simulink model "suspend_kamotu_kato3"  (R2020b)
settings: Solver=ode15s  StartTime=0.0  StopTime=100  FixedStep=0.0001  MaxStep=0.001
settings Model: Creator=iketa  LastModifiedBy=kt012
settings DebuggingCC: ArithmeticOperatorsInVariantConditions=warning
settings SFSimCC: CustomCodeUndefinedFunction=UseInterfaceOnly

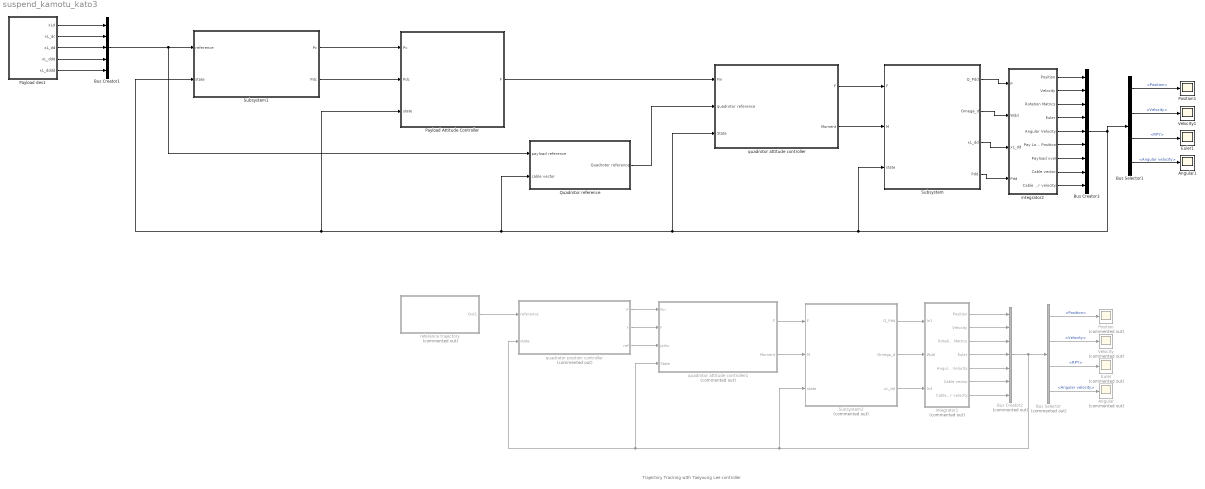
== system suspend_kamotu_kato3 ==
  note: Trajectory Tracking with Taeyoung Lee controller
  Angular : Scope  Commented=on
  Angular1 : Scope
  Bus Creator1 : BusCreator  Inputs=5
  Bus Creator2 : BusCreator  Commented=on  Inputs=7
  Bus Creator3 : BusCreator  Inputs=9
  Bus Selector : BusSelector  Commented=on  OutputSignals=Position,Velocity,RPY,Angular velocity
  Bus Selector1 : BusSelector  OutputSignals=Position,Velocity,RPY,Angular velocity
  Euler : Scope  Commented=on
  Euler1 : Scope
  Payload Attitude Controller : Subsystem
  Payload des1 : MATLAB Function  TreatAsAtomicUnit=on
  Position : Scope  Commented=on
  Position1 : Scope
  Quadrotor reference : Subsystem
  Subsystem : Subsystem
  Subsystem1 : Subsystem
  Subsystem2 : Subsystem  Commented=on
  Velocity : Scope  Commented=on
  Velocity1 : Scope
  integrator1 : Subsystem  Commented=on
  integrator2 : Subsystem
  quadrotor attitude controller : Subsystem
  quadrotor attitude controller1 : Subsystem  Commented=on
  quadrotor position controller : Subsystem  Commented=on
  reference trajectory : Subsystem  Commented=on
  wires:
  Subsystem/1(Q_Pdd) -> integrator2/1(P)
  Subsystem/2(Omega_d) -> integrator2/2(Wdd)
  Subsystem/3(xL_dd) -> integrator2/3(xL_dd)
  Payload Attitude Controller/1(F) -> quadrotor attitude controller/1(Fin)
  quadrotor attitude controller/2(Moment) -> Subsystem/2(M)
  quadrotor attitude controller/1(F) -> Subsystem/1(F)
  Payload des1/4(xL_ddd) -> Bus Creator1/4
  Payload des1/3(xL_dd) -> Bus Creator1/3
  Payload des1/2(xL_dc) -> Bus Creator1/2
  Payload des1/1(xLd) -> Bus Creator1/1
  Bus Creator1/1 -> Quadrotor reference/1(payload reference), Subsystem1/1(reference)
  Subsystem1/1(Pc) -> Payload Attitude Controller/1(Pc)
  Subsystem1/2(Pdc) -> Payload Attitude Controller/2(Pdc)
  quadrotor attitude controller1/1(F) -> Subsystem2/1(F)
  quadrotor attitude controller1/2(Moment) -> Subsystem2/2(M)
  integrator1/6(Cable vector) -> Bus Creator2/6
  integrator1/5(Angular Velocity) -> Bus Creator2/5
  Subsystem2/3(xL_dd) -> integrator1/3(In3)
  integrator1/2(Velocity) -> Bus Creator2/2
  integrator1/3(Rotation Matrics) -> Bus Creator2/3
  Bus Creator2/1 -> quadrotor position controller/2(state), quadrotor attitude controller1/4(State), Subsystem2/3(state), Bus Selector/1
  integrator1/1(Position) -> Bus Creator2/1
  Subsystem2/2(Omega_d) -> integrator1/2(Wdd)
  integrator1/7(Cable vector velocity) -> Bus Creator2/7
  Subsystem2/1(Q_Pdd) -> integrator1/1(In1)
  quadrotor position controller/1(F) -> quadrotor attitude controller1/1(Fin)
  quadrotor position controller/3(ref) -> quadrotor attitude controller1/3(jarkc)
  quadrotor position controller/2(f) -> quadrotor attitude controller1/2(f)
  Bus Selector/1 -> Position/1  "<Position>"
  Bus Selector/2 -> Velocity/1  "<Velocity>"
  Bus Selector/3 -> Euler/1  "<RPY>"
  integrator1/4(Euler) -> Bus Creator2/4
  Bus Selector/4 -> Angular/1  "<Angular velocity>"
  reference trajectory/1(Out1) -> quadrotor position controller/1(reference)
  Payload des1/5(xL_dddd) -> Bus Creator1/5
  Quadrotor reference/1(Quadrotor reference) -> quadrotor attitude controller/2(quadrotor reference)
  Bus Selector1/1 -> Position1/1  "<Position>"
  Bus Selector1/2 -> Velocity1/1  "<Velocity>"
  Bus Selector1/3 -> Euler1/1  "<RPY>"
  Bus Selector1/4 -> Angular1/1  "<Angular velocity>"
  integrator2/4(Euler) -> Bus Creator3/4
  integrator2/2(Velocity) -> Bus Creator3/2
  integrator2/5(Angular Velocity) -> Bus Creator3/5
  integrator2/3(Rotation Matrics) -> Bus Creator3/3
  integrator2/1(Position) -> Bus Creator3/1
  integrator2/9(Cable vector velocity) -> Bus Creator3/9
  Bus Creator3/1 -> Bus Selector1/1, Subsystem/3(state), Subsystem1/2(state), Payload Attitude Controller/3(state), Quadrotor reference/2(cable vector), quadrotor attitude controller/3(State)
  integrator2/8(Cable vector) -> Bus Creator3/8
  Subsystem/4(Pdd) -> integrator2/4(Pdd)
  integrator2/6(Pay Load Position) -> Bus Creator3/6
  integrator2/7(Payload vvel) -> Bus Creator3/7

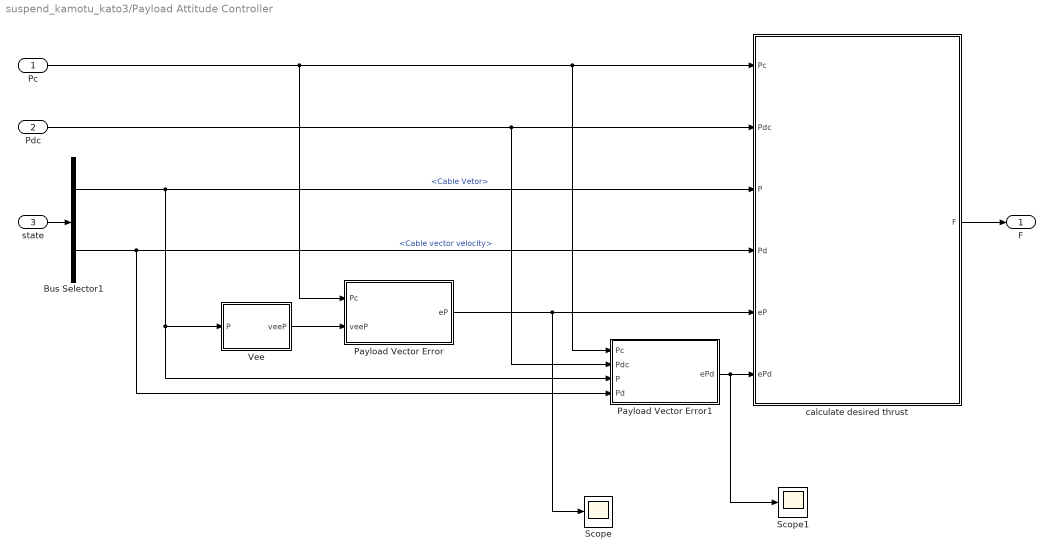
== system suspend_kamotu_kato3/Payload Attitude Controller ==
  Pc : Inport
  Pdc : Inport  Port=2
  state : Inport  Port=3
  Bus Selector1 : BusSelector  OutputSignals=Cable Vetor,Cable vector velocity
  Payload Vector Error : MATLAB Function  TreatAsAtomicUnit=on
  Payload Vector Error1 : MATLAB Function  TreatAsAtomicUnit=on
  Scope : Scope
  Scope1 : Scope
  Vee : MATLAB Function  TreatAsAtomicUnit=on
  calculate desired thrust : MATLAB Function  TreatAsAtomicUnit=on
  F : Outport
  wires:
  Payload Vector Error1/1(ePd) -> Scope1/1, calculate desired thrust/6(ePd)
  state/1 -> Bus Selector1/1
  Pdc/1 -> Payload Vector Error1/2(Pdc), calculate desired thrust/2(Pdc)
  Bus Selector1/1 -> Vee/1(P), Payload Vector Error1/3(P), calculate desired thrust/3(P)  "<Cable Vetor>"
  calculate desired thrust/1(F) -> F/1
  Vee/1(veeP) -> Payload Vector Error/2(veeP)
  Bus Selector1/2 -> Payload Vector Error1/4(Pd), calculate desired thrust/4(Pd)  "<Cable vector velocity>"
  Payload Vector Error/1(eP) -> Scope/1, calculate desired thrust/5(eP)
  Pc/1 -> Payload Vector Error/1(Pc), Payload Vector Error1/1(Pc), calculate desired thrust/1(Pc)

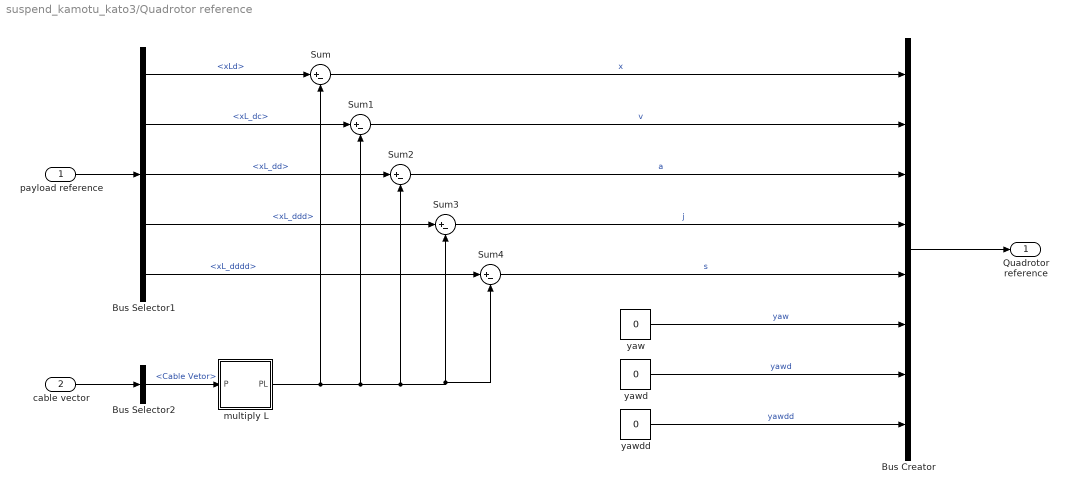
== system suspend_kamotu_kato3/Quadrotor reference ==
  payload reference : Inport
  cable vector : Inport  Port=2
  Bus Creator : BusCreator  Inputs=8
  Bus Selector1 : BusSelector  OutputSignals=xLd,xL_dc,xL_dd,xL_ddd,xL_dddd
  Bus Selector2 : BusSelector  OutputSignals=Cable Vetor
  Sum{,1..4} (5 alike) : Sum  Inputs=|+-
  multiply L : MATLAB Function  TreatAsAtomicUnit=on
  yaw : Constant  Value=0
  yawd : Constant  Value=0
  yawdd : Constant  Value=0
  Quadrotor reference : Outport
  wires:
  Bus Selector1/2 -> Sum1/1  "<xL_dc>"
  multiply L/1(PL) -> Sum4/2, Sum3/2, Sum2/2, Sum1/2, Sum/2
  Sum1/1 -> Bus Creator/2  "v"
  cable vector/1 -> Bus Selector2/1
  Bus Selector1/4 -> Sum3/1  "<xL_ddd>"
  Bus Selector1/1 -> Sum/1  "<xLd>"
  payload reference/1 -> Bus Selector1/1
  Bus Selector1/5 -> Sum4/1  "<xL_dddd>"
  Bus Selector1/3 -> Sum2/1  "<xL_dd>"
  Bus Selector2/1 -> multiply L/1(P)  "<Cable Vetor>"
  Sum2/1 -> Bus Creator/3  "a"
  Sum/1 -> Bus Creator/1  "x"
  Sum3/1 -> Bus Creator/4  "j"
  Sum4/1 -> Bus Creator/5  "s"
  Bus Creator/1 -> Quadrotor reference/1
  yaw/1 -> Bus Creator/6  "yaw"
  yawd/1 -> Bus Creator/7  "yawd"
  yawdd/1 -> Bus Creator/8  "yawdd"

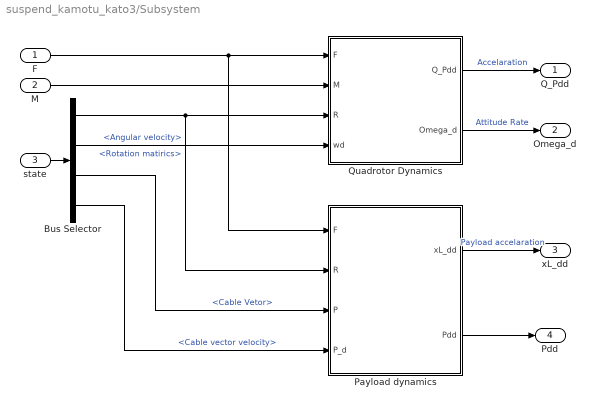
== system suspend_kamotu_kato3/Subsystem ==
  F : Inport
  M : Inport  Port=2
  state : Inport  Port=3
  Bus Selector : BusSelector  OutputSignals=Rotation matirics,Angular velocity,Cable Vetor,Cable vector velocity
  Payload dynamics : MATLAB Function  TreatAsAtomicUnit=on
  Quadrotor Dynamics : MATLAB Function  TreatAsAtomicUnit=on
  Q_Pdd : Outport
  Omega_d : Outport  Port=2
  xL_dd : Outport  Port=3
  Pdd : Outport  Port=4
  wires:
  Payload dynamics/1(xL_dd) -> xL_dd/1  "Payload accelaration"
  Bus Selector/3 -> Payload dynamics/3(P)  "<Cable Vetor>"
  F/1 -> Quadrotor Dynamics/1(F), Payload dynamics/1(F)
  Quadrotor Dynamics/2(Omega_d) -> Omega_d/1  "Attitude Rate"
  Quadrotor Dynamics/1(Q_Pdd) -> Q_Pdd/1  "Accelaration"
  state/1 -> Bus Selector/1
  Bus Selector/1 -> Quadrotor Dynamics/3(R), Payload dynamics/2(R)  "<Rotation matirics>"
  Bus Selector/4 -> Payload dynamics/4(P_d)  "<Cable vector velocity>"
  M/1 -> Quadrotor Dynamics/2(M)
  Bus Selector/2 -> Quadrotor Dynamics/4(wd)  "<Angular velocity>"
  Payload dynamics/2(Pdd) -> Pdd/1

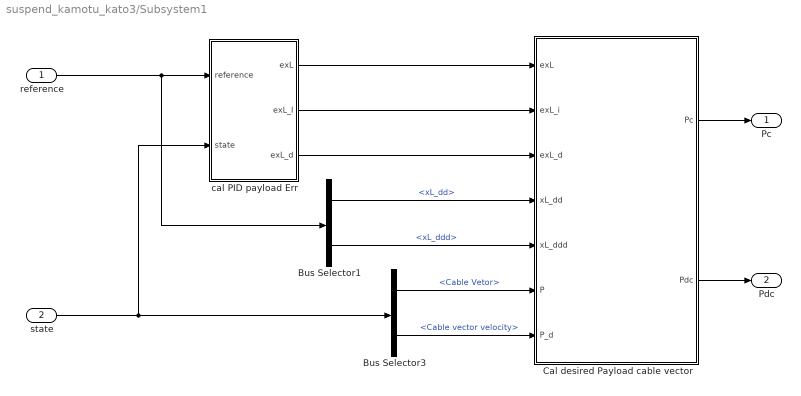
== system suspend_kamotu_kato3/Subsystem1 ==
  reference : Inport
  state : Inport  Port=2
  Bus Selector1 : BusSelector  OutputSignals=xL_dd,xL_ddd
  Bus Selector3 : BusSelector  OutputSignals=Cable Vetor,Cable vector velocity
  Cal desired Payload cable vector : MATLAB Function  TreatAsAtomicUnit=on
  cal PID payload Err : Subsystem
  Pc : Outport
  Pdc : Outport  Port=2
  wires:
  state/1 -> Bus Selector3/1, cal PID payload Err/2(state)
  Bus Selector3/2 -> Cal desired Payload cable vector/7(P_d)  "<Cable vector velocity>"
  Bus Selector3/1 -> Cal desired Payload cable vector/6(P)  "<Cable Vetor>"
  Cal desired Payload cable vector/1(Pc) -> Pc/1
  Cal desired Payload cable vector/2(Pdc) -> Pdc/1
  reference/1 -> Bus Selector1/1, cal PID payload Err/1(reference)
  cal PID payload Err/1(exL) -> Cal desired Payload cable vector/1(exL)
  cal PID payload Err/2(exL_I) -> Cal desired Payload cable vector/2(exL_i)
  cal PID payload Err/3(exL_d) -> Cal desired Payload cable vector/3(exL_d)
  Bus Selector1/1 -> Cal desired Payload cable vector/4(xL_dd)  "<xL_dd>"
  Bus Selector1/2 -> Cal desired Payload cable vector/5(xL_ddd)  "<xL_ddd>"

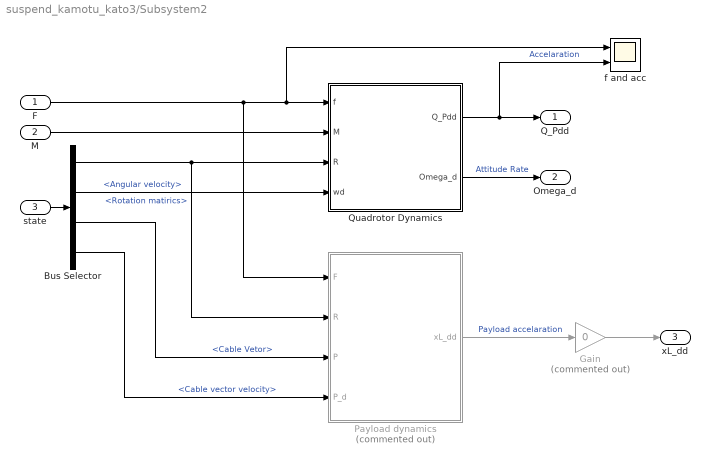
== system suspend_kamotu_kato3/Subsystem2 ==
  F : Inport
  M : Inport  Port=2
  state : Inport  Port=3
  Bus Selector : BusSelector  OutputSignals=Rotation matirics,Angular velocity,Cable Vetor,Cable vector velocity
  Gain : Gain  Commented=on  Gain=0
  Payload dynamics : MATLAB Function  Commented=on  TreatAsAtomicUnit=on
  Quadrotor Dynamics : MATLAB Function  TreatAsAtomicUnit=on
  f and acc : Scope  NumInputPorts=2
  Q_Pdd : Outport
  Omega_d : Outport  Port=2
  xL_dd : Outport  Port=3
  wires:
  Payload dynamics/1(xL_dd) -> Gain/1  "Payload accelaration"
  Bus Selector/3 -> Payload dynamics/3(P)  "<Cable Vetor>"
  F/1 -> Payload dynamics/1(F), f and acc/1, Quadrotor Dynamics/1(f)
  Quadrotor Dynamics/2(Omega_d) -> Omega_d/1  "Attitude Rate"
  Quadrotor Dynamics/1(Q_Pdd) -> f and acc/2, Q_Pdd/1  "Accelaration"
  state/1 -> Bus Selector/1
  Bus Selector/1 -> Payload dynamics/2(R), Quadrotor Dynamics/3(R)  "<Rotation matirics>"
  Bus Selector/4 -> Payload dynamics/4(P_d)  "<Cable vector velocity>"
  M/1 -> Quadrotor Dynamics/2(M)
  Bus Selector/2 -> Quadrotor Dynamics/4(wd)  "<Angular velocity>"
  Gain/1 -> xL_dd/1

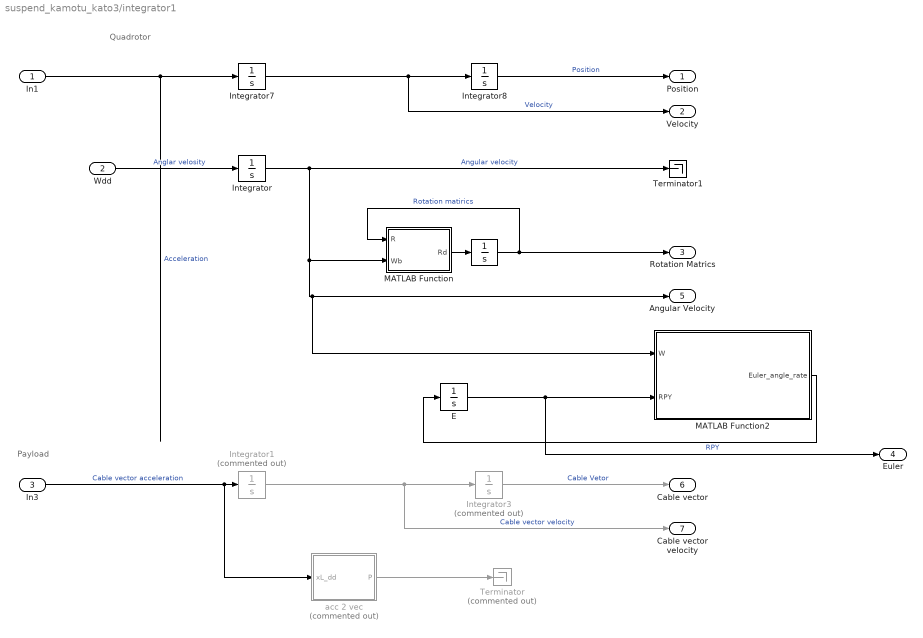
== system suspend_kamotu_kato3/integrator1 ==
  note: Quadrotor
  note: Payload
  In1 : Inport
  Wdd : Inport  Port=2
  In3 : Inport  Port=3
  " " : Integrator  InitialCondition=[1 0 0; 0 1 0; 0 0 1];  ContinuousStateAttributes="\"\""
  E : Integrator  InitialCondition=[0 0 0];
  Integrator : Integrator  InitialCondition=[0 ;0;0];
  Integrator1 : Integrator  Commented=on  InitialCondition=[0;0;0]
  Integrator3 : Integrator  Commented=on  InitialCondition=[0;0;-1]
  Integrator7 : Integrator  InitialCondition=[0;0;0]
  Integrator8 : Integrator  InitialCondition=[0;0;0];
  MATLAB Function : MATLAB Function  TreatAsAtomicUnit=on
  MATLAB Function2 : MATLAB Function  TreatAsAtomicUnit=on
  Terminator : Terminator  Commented=on
  Terminator1 : Terminator
  acc 2 vec : MATLAB Function  Commented=on  TreatAsAtomicUnit=on
  Position : Outport
  Velocity : Outport  Port=2
  Rotation Matrics : Outport  Port=3
  Euler : Outport  Port=4
  Angular Velocity : Outport  Port=5
  Cable vector : Outport  Port=6
  Cable vector velocity : Outport  Port=7
  wires:
  In3/1 -> Integrator1/1, acc 2 vec/1(xL_dd)  "Cable vector acceleration"
  Integrator1/1 -> Integrator3/1, Cable vector velocity/1  "Cable vector velocity"
  acc 2 vec/1(P) -> Terminator/1
  Integrator3/1 -> Cable vector/1  "Cable Vetor"
  Integrator7/1 -> Velocity/1, Integrator8/1  "Velocity"
  Integrator8/1 -> Position/1  "Position"
  In1/1 -> Integrator7/1  "Acceleration"
  MATLAB Function/1(Rd) -> " "/1
  Wdd/1 -> Integrator/1  "Anglar velosity"
  " "/1 -> Rotation Matrics/1, MATLAB Function/1(R)  "Rotation matirics"
  Integrator/1 -> MATLAB Function/2(Wb), MATLAB Function2/1(W), Angular Velocity/1, Terminator1/1  "Angular velocity"
  E/1 -> MATLAB Function2/2(RPY), Euler/1  "RPY"
  MATLAB Function2/1(Euler_angle_rate) -> E/1

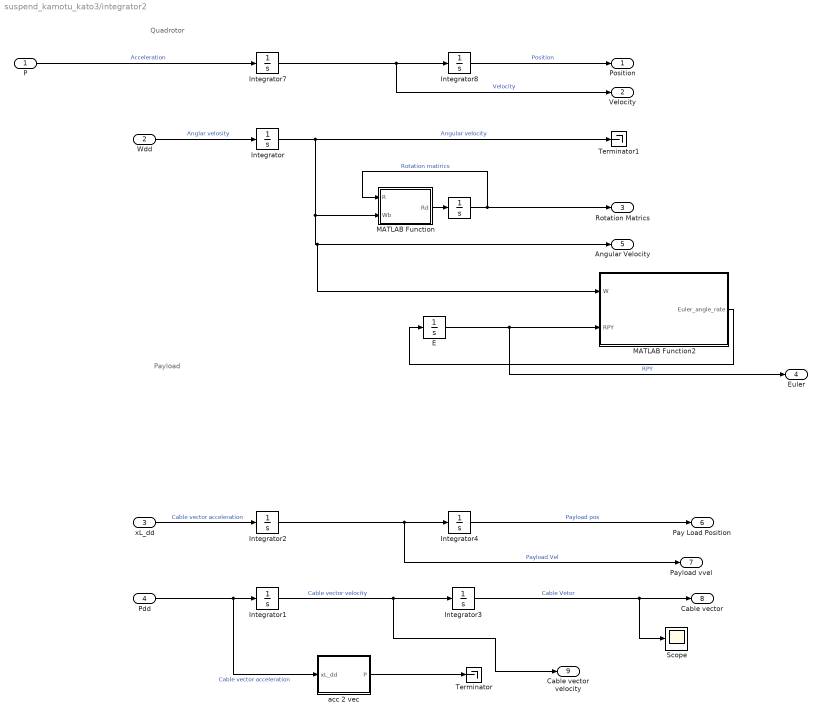
== system suspend_kamotu_kato3/integrator2 ==
  note: Quadrotor
  note: Payload
  P : Inport
  Wdd : Inport  Port=2
  xL_dd : Inport  Port=3
  Pdd : Inport  Port=4
  " " : Integrator  InitialCondition=[1 0 0; 0 1 0; 0 0 1];  ContinuousStateAttributes="\"\""
  E : Integrator  InitialCondition=[0 0 0];
  Integrator : Integrator  InitialCondition=[0 ;0;0];
  Integrator1 : Integrator  InitialCondition=[0;0;0]
  Integrator2 : Integrator  InitialCondition=[0;0;0]
  Integrator3 : Integrator  InitialCondition=[0;0;-1]
  Integrator4 : Integrator  InitialCondition=[0;0;-1]
  Integrator7 : Integrator  InitialCondition=[0;0;0]
  Integrator8 : Integrator  InitialCondition=[0;0;0.1];
  MATLAB Function : MATLAB Function  TreatAsAtomicUnit=on
  MATLAB Function2 : MATLAB Function  TreatAsAtomicUnit=on
  Scope : Scope
  Terminator : Terminator
  Terminator1 : Terminator
  acc 2 vec : MATLAB Function  TreatAsAtomicUnit=on
  Position : Outport
  Velocity : Outport  Port=2
  Rotation Matrics : Outport  Port=3
  Euler : Outport  Port=4
  Angular Velocity : Outport  Port=5
  Pay Load Position : Outport  Port=6
  Payload vvel : Outport  Port=7
  Cable vector : Outport  Port=8
  Cable vector velocity : Outport  Port=9
  wires:
  Pdd/1 -> acc 2 vec/1(xL_dd), Integrator1/1  "Cable vector acceleration"
  Integrator1/1 -> Integrator3/1, Cable vector velocity/1  "Cable vector velocity"
  acc 2 vec/1(P) -> Terminator/1
  Integrator3/1 -> Scope/1, Cable vector/1  "Cable Vetor"
  Integrator7/1 -> Velocity/1, Integrator8/1  "Velocity"
  Integrator8/1 -> Position/1  "Position"
  P/1 -> Integrator7/1  "Acceleration"
  MATLAB Function/1(Rd) -> " "/1
  Wdd/1 -> Integrator/1  "Anglar velosity"
  " "/1 -> Rotation Matrics/1, MATLAB Function/1(R)  "Rotation matirics"
  Integrator/1 -> MATLAB Function/2(Wb), MATLAB Function2/1(W), Angular Velocity/1, Terminator1/1  "Angular velocity"
  E/1 -> MATLAB Function2/2(RPY), Euler/1  "RPY"
  MATLAB Function2/1(Euler_angle_rate) -> E/1
  xL_dd/1 -> Integrator2/1  "Cable vector acceleration"
  Integrator2/1 -> Payload vvel/1, Integrator4/1  "Payload Vel"
  Integrator4/1 -> Pay Load Position/1  "Payload pos"

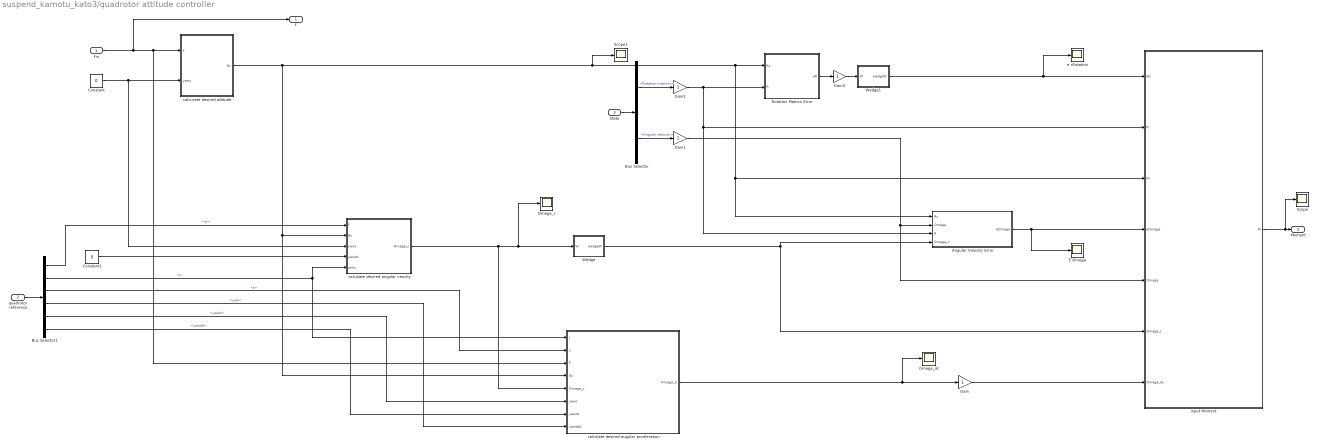
== system suspend_kamotu_kato3/quadrotor attitude controller ==
  Fin : Inport
  quadrotor reference : Inport  Port=2
  State : Inport  Port=3
  Angular Velocity Error : MATLAB Function  TreatAsAtomicUnit=on
  Bus Selector : BusSelector  OutputSignals=Rotation matirics,Angular velocity
  Bus Selector1 : BusSelector  OutputSignals=a,j,s,yaw,yawd,yawdd
  Constant : Constant  Value=0
  Constant1 : Constant  Value=0
  E Omega : Scope
  Gain{,1..3} (4 alike) : Gain
  Omega_c : Scope
  Omega_dc : Scope
  Rotation Matrics Error : MATLAB Function  TreatAsAtomicUnit=on
  Scope : Scope
  Scope1 : Scope
  Wedge : MATLAB Function  TreatAsAtomicUnit=on
  Wedge1 : MATLAB Function  TreatAsAtomicUnit=on
  calculate desired angular veocity : MATLAB Function  TreatAsAtomicUnit=on
  calculate desired augular acceleration : MATLAB Function  TreatAsAtomicUnit=on
  calcurate desired attitude : MATLAB Function  TreatAsAtomicUnit=on
  e rRotation : Scope
  input Moment : MATLAB Function  TreatAsAtomicUnit=on
  F : Outport
  Moment : Outport  Port=2
  wires:
  Gain3/1 -> Wedge1/1(W)
  Gain2/1 -> Angular Velocity Error/3(R), input Moment/2(R), Rotation Matrics Error/2(R)
  Wedge/1(wedgeW) -> Angular Velocity Error/4(Omega_c), input Moment/6(Omega_c)
  calculate desired augular acceleration/1(Omega_d) -> Omega_dc/1, Gain/1
  calculate desired angular veocity/1(Omega_c) -> Omega_c/1, Wedge/1(W), calculate desired augular acceleration/5(Omega_c)
  input Moment/1(M) -> Scope/1, Moment/1
  Bus Selector1/5 -> calculate desired augular acceleration/6(yawc)  "<yawd>"
  Rotation Matrics Error/1(eR) -> Gain3/1
  Gain/1 -> input Moment/7(Omega_dc)
  Bus Selector1/1 -> calculate desired angular veocity/1(F)  "<a>"
  Bus Selector1/4 -> calculate desired augular acceleration/8(yawddc)  "<yaw>"
  Bus Selector1/3 -> calculate desired augular acceleration/2(s)  "<s>"
  Bus Selector/1 -> Gain2/1  "<Rotation matirics>"
  quadrotor reference/1 -> Bus Selector1/1
  State/1 -> Bus Selector/1
  calcurate desired attitude/1(Rc) -> calculate desired augular acceleration/4(Rc), calculate desired angular veocity/2(Rc), Angular Velocity Error/1(Rc), input Moment/3(Rc), Rotation Matrics Error/1(Rc), Scope1/1
  Bus Selector1/6 -> calculate desired augular acceleration/7(yawdc)  "<yawdd>"
  Fin/1 -> F/1, calculate desired augular acceleration/3(F), calcurate desired attitude/1(F)
  Bus Selector1/2 -> calculate desired angular veocity/5(jarkc), calculate desired augular acceleration/1(j)  "<j>"
  Constant/1 -> calcurate desired attitude/2(yawc), calculate desired angular veocity/3(yawc)
  Constant1/1 -> calculate desired angular veocity/4(yawdc)
  Bus Selector/2 -> Gain1/1  "<Angular velocity>"
  Wedge1/1(wedgeW) -> e rRotation/1, input Moment/1(eR)
  Gain1/1 -> input Moment/5(Omega), Angular Velocity Error/2(Omega)
  Angular Velocity Error/1(eOmega) -> E Omega/1, input Moment/4(eOmega)

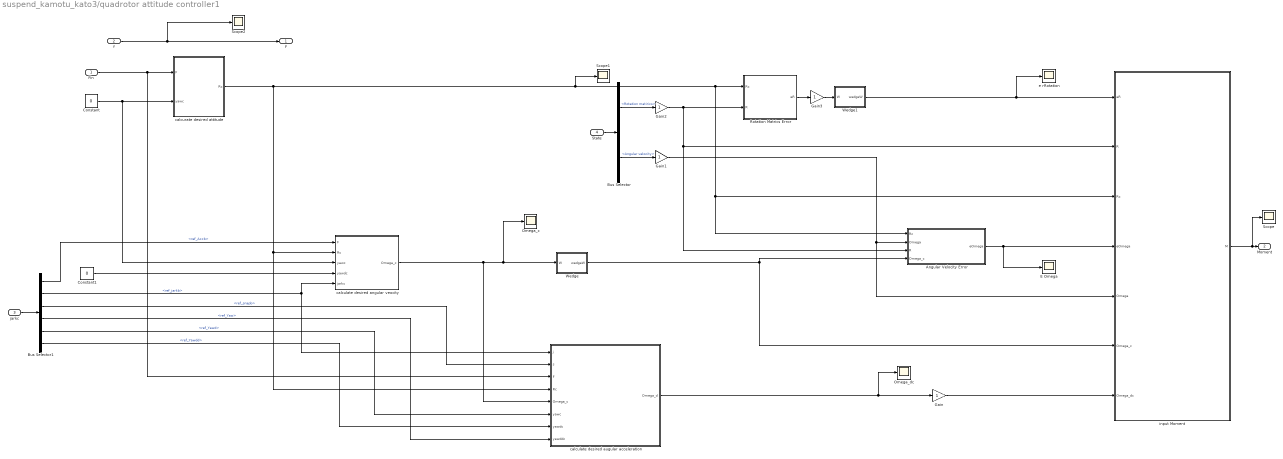
== system suspend_kamotu_kato3/quadrotor attitude controller1 ==
  Fin : Inport
  f : Inport  Port=2
  jarkc : Inport  Port=3
  State : Inport  Port=4
  Angular Velocity Error : MATLAB Function  TreatAsAtomicUnit=on
  Bus Selector : BusSelector  OutputSignals=Rotation matirics,Angular velocity
  Bus Selector1 : BusSelector  OutputSignals=ref_Accb,ref_jarkb,ref_snapb,ref_Yaw,ref_Yawd,ref_Yawdd
  Constant : Constant  Value=0
  Constant1 : Constant  Value=0
  E Omega : Scope
  Gain{,1..3} (4 alike) : Gain
  Omega_c : Scope
  Omega_dc : Scope
  Rotation Matrics Error : MATLAB Function  TreatAsAtomicUnit=on
  Scope : Scope
  Scope1 : Scope
  Scope2 : Scope
  Wedge : MATLAB Function  TreatAsAtomicUnit=on
  Wedge1 : MATLAB Function  TreatAsAtomicUnit=on
  calculate desired angular veocity : MATLAB Function  TreatAsAtomicUnit=on
  calculate desired augular acceleration : MATLAB Function  TreatAsAtomicUnit=on
  calcurate desired attitude : MATLAB Function  TreatAsAtomicUnit=on
  e rRotation : Scope
  input Moment : MATLAB Function  TreatAsAtomicUnit=on
  F : Outport
  Moment : Outport  Port=2
  wires:
  calcurate desired attitude/1(Rc) -> calculate desired augular acceleration/4(Rc), calculate desired angular veocity/2(Rc), Angular Velocity Error/1(Rc), input Moment/3(Rc), Rotation Matrics Error/1(Rc), Scope1/1
  Constant1/1 -> calculate desired angular veocity/4(yawdc)
  Bus Selector/2 -> Gain1/1  "<Angular velocity>"
  calculate desired angular veocity/1(Omega_c) -> Omega_c/1, Wedge/1(W), calculate desired augular acceleration/5(Omega_c)
  State/1 -> Bus Selector/1
  Bus Selector/1 -> Gain2/1  "<Rotation matirics>"
  Angular Velocity Error/1(eOmega) -> E Omega/1, input Moment/4(eOmega)
  Rotation Matrics Error/1(eR) -> Gain3/1
  Constant/1 -> calcurate desired attitude/2(yawc), calculate desired angular veocity/3(yawc)
  Fin/1 -> calculate desired augular acceleration/3(F), calcurate desired attitude/1(F)
  jarkc/1 -> Bus Selector1/1
  Wedge/1(wedgeW) -> Angular Velocity Error/4(Omega_c), input Moment/6(Omega_c)
  Wedge1/1(wedgeW) -> e rRotation/1, input Moment/1(eR)
  Bus Selector1/2 -> calculate desired angular veocity/5(jarkc), calculate desired augular acceleration/1(j)  "<ref_jarkb>"
  Bus Selector1/3 -> calculate desired augular acceleration/2(s)  "<ref_snapb>"
  Bus Selector1/5 -> calculate desired augular acceleration/6(yawc)  "<ref_Yawd>"
  Bus Selector1/6 -> calculate desired augular acceleration/7(yawdc)  "<ref_Yawdd>"
  calculate desired augular acceleration/1(Omega_d) -> Omega_dc/1, Gain/1
  Bus Selector1/4 -> calculate desired augular acceleration/8(yawddc)  "<ref_Yaw>"
  input Moment/1(M) -> Scope/1, Moment/1
  Gain/1 -> input Moment/7(Omega_dc)
  f/1 -> Scope2/1, F/1
  Gain2/1 -> Angular Velocity Error/3(R), input Moment/2(R), Rotation Matrics Error/2(R)
  Gain1/1 -> input Moment/5(Omega), Angular Velocity Error/2(Omega)
  Bus Selector1/1 -> calculate desired angular veocity/1(F)  "<ref_Accb>"
  Gain3/1 -> Wedge1/1(W)

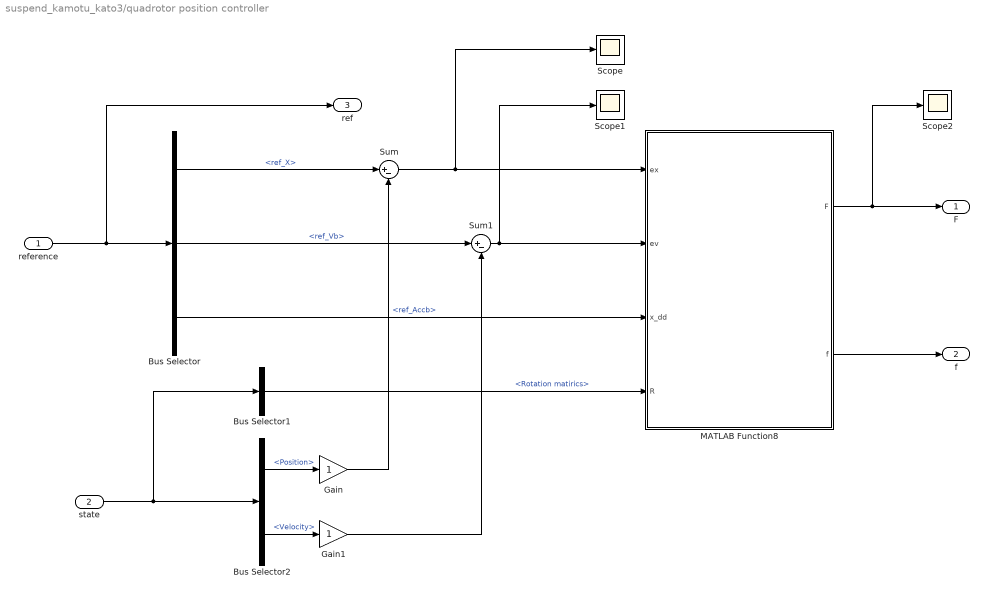
== system suspend_kamotu_kato3/quadrotor position controller ==
  reference : Inport
  state : Inport  Port=2
  Bus Selector : BusSelector  OutputSignals=ref_X,ref_Vb,ref_Accb
  Bus Selector1 : BusSelector  OutputSignals=Rotation matirics
  Bus Selector2 : BusSelector  OutputSignals=Position,Velocity
  Gain : Gain
  Gain1 : Gain
  MATLAB Function8 : MATLAB Function
  Scope : Scope
  Scope1 : Scope
  Scope2 : Scope
  Sum : Sum  Inputs=|+-
  Sum1 : Sum  Inputs=|+-
  F : Outport
  f : Outport  Port=2
  ref : Outport  Port=3
  wires:
  Bus Selector/2 -> Sum1/1  "<ref_Vb>"
  reference/1 -> ref/1, Bus Selector/1
  Sum/1 -> MATLAB Function8/1(ex), Scope/1
  MATLAB Function8/1(F) -> Scope2/1, F/1
  Bus Selector1/1 -> MATLAB Function8/4(R)  "<Rotation matirics>"
  Sum1/1 -> MATLAB Function8/2(ev), Scope1/1
  Bus Selector/3 -> MATLAB Function8/3(x_dd)  "<ref_Accb>"
  Bus Selector/1 -> Sum/1  "<ref_X>"
  state/1 -> Bus Selector1/1, Bus Selector2/1
  Bus Selector2/1 -> Gain/1  "<Position>"
  Bus Selector2/2 -> Gain1/1  "<Velocity>"
  MATLAB Function8/2(f) -> f/1
  Gain/1 -> Sum/2
  Gain1/1 -> Sum1/2

== system suspend_kamotu_kato3/reference trajectory ==
  Bus Creator3 : BusCreator  Inputs=8
  Clock2 : Clock
      settings: Decimation=100
  Constant3 : Constant  Value=50
  Constant4 : Constant
  Reference Trajectory : MATLAB Function  TreatAsAtomicUnit=on
  Out1 : Outport
  wires:
  Reference Trajectory/1(ref_X) -> Bus Creator3/1
  Constant4/1 -> Reference Trajectory/3(r)
  Reference Trajectory/6(ref_Yaw) -> Bus Creator3/6
  Reference Trajectory/2(ref_Vb) -> Bus Creator3/2
  Reference Trajectory/4(ref_jarkb) -> Bus Creator3/4
  Constant3/1 -> Reference Trajectory/2(T)
  Reference Trajectory/5(ref_snapb) -> Bus Creator3/5
  Clock2/1 -> Reference Trajectory/1(t)
  Reference Trajectory/3(ref_Accb) -> Bus Creator3/3
  Reference Trajectory/7(ref_Yawd) -> Bus Creator3/7
  Reference Trajectory/8(ref_Yawdd) -> Bus Creator3/8
  Bus Creator3/1 -> Out1/1

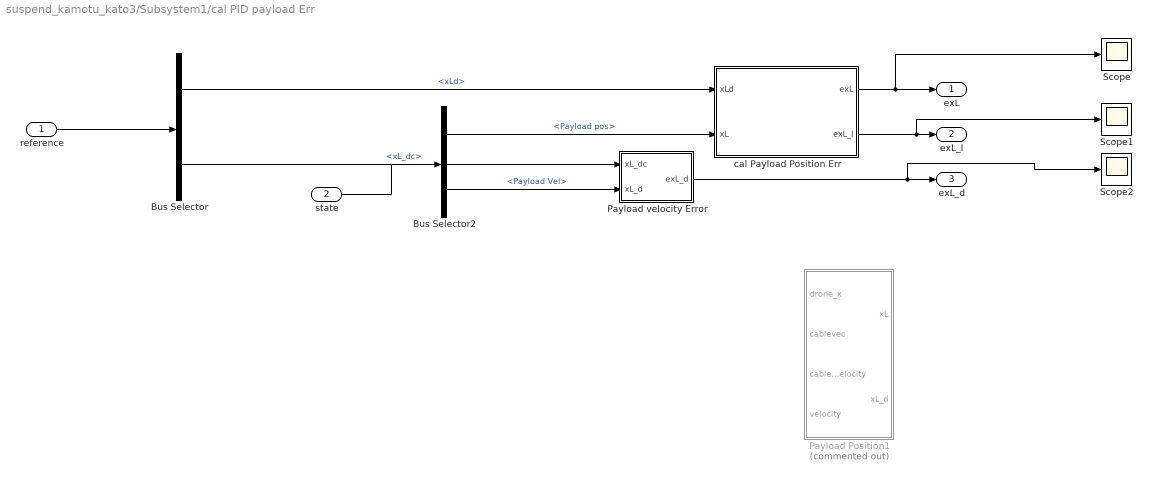
== system suspend_kamotu_kato3/Subsystem1/cal PID payload Err ==
  reference : Inport
  state : Inport  Port=2
  Bus Selector : BusSelector  OutputSignals=xLd,xL_dc
  Bus Selector2 : BusSelector  OutputSignals=Payload pos,Payload Vel
  Payload Position1 : MATLAB Function  Commented=on  TreatAsAtomicUnit=on
  Payload velocity Error : MATLAB Function  TreatAsAtomicUnit=on
  Scope : Scope
  Scope1 : Scope
  Scope2 : Scope
  cal Payload Position Err : Subsystem
  exL : Outport
  exL_I : Outport  Port=2
  exL_d : Outport  Port=3
  wires:
  state/1 -> Bus Selector2/1
  Bus Selector/1 -> cal Payload Position Err/1(xLd)  "<xLd>"
  Bus Selector/2 -> Payload velocity Error/1(xL_dc)  "<xL_dc>"
  Payload velocity Error/1(exL_d) -> Scope2/1, exL_d/1
  cal Payload Position Err/1(exL) -> Scope/1, exL/1
  cal Payload Position Err/2(exL_I) -> Scope1/1, exL_I/1
  reference/1 -> Bus Selector/1
  Bus Selector2/1 -> cal Payload Position Err/2(xL)  "<Payload pos>"
  Bus Selector2/2 -> Payload velocity Error/2(xL_d)  "<Payload Vel>"

== system suspend_kamotu_kato3/Subsystem1/cal PID payload Err/cal Payload Position Err ==
  xLd : Inport
  xL : Inport  Port=2
  Integrator : Integrator
  Payload Positon Error : MATLAB Function  TreatAsAtomicUnit=on
  exL : Outport
  exL_I : Outport  Port=2
  wires:
  Payload Positon Error/1(exL) -> exL/1, Integrator/1
  xLd/1 -> Payload Positon Error/1(xLd)
  Integrator/1 -> exL_I/1
  xL/1 -> Payload Positon Error/2(xL)

== matlab function suspend_kamotu_kato3/quadrotor attitude controller1/calcurate desired attitude ==
  data: F input; Rc output; yawc input
function Rc = fcn(F, yawc)

b3c = F/norm(F);
c1c = [cos(yawc); sin(yawc); 0];
c2c = [-sin(yawc); cos(yawc); 0];

b1c = cross(cross(b3c, c1c)/norm(cross(b3c, c1c)), b3c);
b2c = cross(b3c, c1c)/norm(cross(b3c, c1c));
Rc = [b1c'; b2c'; b3c'];

== matlab function suspend_kamotu_kato3/quadrotor attitude controller/Angular Velocity Error ==
  data: Rc input; Omega input; R input; Omega_c input; eOmega output
function eOmega = fcn(Rc, Omega,R, Omega_c)

eOmega = Omega - R'*Rc*Omega_c;
% eOmega = Omega - Omega_c;

== matlab function suspend_kamotu_kato3/quadrotor attitude controller/Rotation Matrics Error ==
  data: Rc input; R input; eR output
function eR = fcn(Rc, R)

eR = (Rc'*R - R'*Rc)/2;

== matlab function suspend_kamotu_kato3/quadrotor attitude controller1/input Moment ==
  data: eR input; R input; Rc input; eOmega input; Omega input; Omega_c input; Omega_dc input; M output
function M = fcn(eR, R, Rc, eOmega, Omega, Omega_c, Omega_dc)

p = paramdef;
Omegavee = [0 -Omega(3) Omega(2); Omega(3) 0 -Omega(1); -Omega(2) Omega(1) 0];
% 角速度入力の時
% M = -p.kR*eR + Omega_c; %- p.I*(cross(Omegavee, R'*Rc*Omega_c) - R'*Rc*Omega_d);

% トルク入力の時
M = -p.kR*eR - p.kOmega*eOmega + cross(Omega, p.I*Omega) - p.I*(Omegavee*R'*Rc*Omega_c - R'*Rc*Omega_dc);
% M = -p.kR*eR - p.kOmega*eOmega + p.I*Omega_dc;

== matlab function suspend_kamotu_kato3/integrator2/MATLAB Function ==
  data: R input; Rd output; Wb input
function Rd = fcn(R, Wb)
wx = Wb(1);
wy = Wb(2);
wz = Wb(3);
Wb = [ 0    -wz   wy;
       wz    0   -wx;
      -wy    wx   0];
Rd = R * Wb;

== matlab function suspend_kamotu_kato3/quadrotor attitude controller/Wedge ==
  data: W input; wedgeW output
function wedgeW= fcn(W)
wedgeW = zeros(3, 1);
wedgeW(1) = W(3, 2);
wedgeW(2) = W(1, 3);
wedgeW(3) = W(2, 1);

== matlab function suspend_kamotu_kato3/integrator2/MATLAB Function2 ==
  data: W input; Euler_angle_rate output; RPY input
function Euler_angle_rate = fcn(W, RPY)
roll = RPY(1);
pitch = RPY(2);
yaw = RPY(3);
rollS = sin(roll); rollC = cos(roll);           
pitchS = sin(pitch); pitchC = cos(pitch);       


Euler_angle_rate = pinv([1 0 -pitchS;
     0 rollC  pitchC * rollS;
     0 -rollS pitchC * rollC]) * W;

== matlab function suspend_kamotu_kato3/integrator2/acc 2 vec ==
  data: xL_dd input; P output
function P  = fcn(xL_dd)                 
g = 9.8;
P = -(xL_dd + g * [0;0;1])/norm(xL_dd + g * [0;0;1]);%ケーブルベクトル

== matlab function suspend_kamotu_kato3/Payload Attitude Controller/Payload Vector Error ==
  data: Pc input; veeP input; eP output
function eP = fcn(Pc, veeP)

eP = veeP^2 * Pc;

== matlab function suspend_kamotu_kato3/Payload Attitude Controller/Vee ==
  data: P input; veeP output
function veeP= fcn(P)
veeP = [0 -P(3) P(2); P(3) 0 -P(1); -P(2) P(1) 0];

== matlab function suspend_kamotu_kato3/Payload Attitude Controller/Payload Vector Error1 ==
  data: Pc input; Pdc input; P input; ePd output; Pd input
function ePd = fcn(Pc,Pdc, P, Pd)

ePd = Pd - cross(cross(Pc, Pdc), P);

== matlab function suspend_kamotu_kato3/Payload Attitude Controller/calculate desired thrust ==
  data: Pc input; Pdc input; P input; F output; Pd input; eP input; ePd input
function F = fcn( Pc, Pdc, P, Pd, eP, ePd)

p = paramdef;
% ----- input thrust calculation ----
F = p.mQ*p.L * (-p.kp*eP - p.kpd*ePd + dot(P, cross(Pc, Pdc))*cross(P, Pd))-dot(Pc, P)*Pc ;%+ p.mQ*p.L *cross(cross(Pc, Pddc), P);

== matlab function suspend_kamotu_kato3/quadrotor attitude controller/Wedge1 ==
  data: W input; wedgeW output
function wedgeW= fcn(W)
wedgeW = zeros(3, 1);
wedgeW(1) = W(3, 2);
wedgeW(2) = W(1, 3);
wedgeW(3) = W(2, 1);

== matlab function suspend_kamotu_kato3/Subsystem2/Payload dynamics ==
  data: F input; R input; P input; xL_dd output; P_d input
function xL_dd  = fcn(F,R,P,P_d)                 
g = 9.8;
e3 = [0;0;1];
p = paramdef;
f = norm(F);
xL_dd = (dot(P, f*R*e3) -p.mQ*p.L*(dot(P_d,P_d))*P)/(p.mQ + p.mL) - g*e3;

== matlab function suspend_kamotu_kato3/quadrotor attitude controller/calculate desired angular veocity ==
  data: F input; Omega_c output; Rc input; yawc input; yawdc input; jarkc input
function Omega_c = fcn(F, Rc, yawc, yawdc, jarkc)

b1c = zeros(3, 1);b2c = zeros(3, 1);b3c = zeros(3, 1);

b1c = Rc(:, 1);
b2c = Rc(:, 2);

b3c = F/norm(F);
c1c = [cos(yawc); sin(yawc); 0];
c2c = [-sin(yawc) cos(yawc) 0]';

wy = dot(b1c, jarkc) / dot(b3c, F);
wx = - dot(b2c, jarkc) / dot(b3c, F);
wz = (yawdc * dot(c1c, b1c) + wy * dot(c2c, b3c))/norm(cross(c2c, b3c));

ref_W = [wx wy wz];
Omega_c = [0,-wz,wy; wz,0,-wx; -wy,wx,0];

== matlab function suspend_kamotu_kato3/Subsystem1/cal PID payload Err/cal Payload Position Err/Payload Positon Error ==
  data: xLd input; xL input; exL output
function exL = fcn(xLd, xL)

exL = xL - xLd;

== matlab function suspend_kamotu_kato3/Subsystem1/cal PID payload Err/Payload velocity Error ==
  data: xL_dc input; xL_d input; exL_d output
function exL_d = fcn(xL_dc, xL_d)

exL_d = (xL_d - xL_dc);

== matlab function suspend_kamotu_kato3/quadrotor attitude controller1/Wedge ==
  data: W input; wedgeW output
function wedgeW= fcn(W)
wedgeW = zeros(3, 1);
wedgeW(1) = W(3, 2);
wedgeW(2) = W(1, 3);
wedgeW(3) = W(2, 1);

== matlab function suspend_kamotu_kato3/Subsystem1/Cal desired Payload cable vector ==
  data: exL input; exL_i input; Pc output; Pdc output; exL_d input; xL_dd input; xL_ddd input; P input; P_d input
function [Pc,Pdc]= fcn(exL,exL_i,exL_d,xL_dd,xL_ddd,P, P_d)
ez = [0;0;1];
p = paramdef;
A = (p.mQ + p.mL) * (-p.kx .* exL - p.kv .* exL_d - p.ki .* exL_i) + (p.mQ + p.mL) * (xL_dd + p.g * ez) + p.mQ * p.L * (P_d' * P_d) * P;
A_d = (p.mQ + p.mL) * (-p.kx .* exL -p.ki .* exL) + (p.mQ + p.mL) * (xL_ddd + p.g * ez) + 0*p.mQ * p.L * (P_d' * P_d) * P_d;

Pc = - A / norm(A);
Pdc = - A_d / norm(A);

== matlab function suspend_kamotu_kato3/Quadrotor reference/multiply L ==
  data: P input; PL output
function PL = fcn(P)
p = paramdef;

PL = P*p.L;

== matlab function suspend_kamotu_kato3/Payload des1 ==
  data: xLd output; xL_dc output; xL_dd output; xL_ddd output; xL_dddd output
function [xLd,xL_dc,xL_dd,xL_ddd,xL_dddd]= fcn
c = [0;0;0];
T = 50;
r = 1;
w = 2 * pi/T;                                       % 角周波数
xLd = c + r*[sin(w*T); cos(w*T); 0] ;               % 貨物の軌道
xL_dc = r*[w*cos(w*T); -w*sin(w*T); 0];             % 貨物の速度
xL_dd = r*[-w^2*sin(w*T); -w^2*cos(w*T); 0];        % 貨物の加速度
xL_ddd = r*[-w^3*cos(w*T); w^3*sin(w*T); 0];        % 加加速度の軌道
xL_dddd = r*[-w^4*sin(w*T); w^4*cos(w*T); 0];        % 加加加速度の軌道

xLd = c + r*[0; 0; 0];
xL_dc = r*[0; 0; 100];
xL_dd = [0; 0; 9.8];
xL_ddd = r*[0;0; 0];
xL_dddd = r*[0;0; 0];

== matlab function suspend_kamotu_kato3/quadrotor attitude controller1/Wedge1 ==
  data: W input; wedgeW output
function wedgeW= fcn(W)
wedgeW = zeros(3, 1);
wedgeW(1) = W(3, 2);
wedgeW(2) = W(1, 3);
wedgeW(3) = W(2, 1);

== matlab function suspend_kamotu_kato3/quadrotor attitude controller1/calculate desired augular acceleration ==
  data: j input; s input; F input; Omega_d output; Rc input; Omega_c input; yawc input; yawdc input; yawddc input
function Omega_d = fcn(j, s, F,Rc, Omega_c, yawc, yawdc, yawddc)
p = paramdef;
m = p.mQ;
Xc = [cos(yawc); sin(yawc); 0];
Yc = [-sin(yawc); cos(yawc); 0];

Zw = [0;0;1];
Xb = Rc(:, 1);
Yb = Rc(:, 2);
Zb = Rc(:, 3);

Wx = Omega_c(3, 2);
Wy = Omega_c(1, 3);
Wz = Omega_c(2, 1);

c =  Zb'*F;
cd = (Rc*Omega_c*Zw)' * F + Zb'*j;

B1 = c;
C3 = norm(cross(Yc, Zb));
A2 = c;
B3 = -Yc'*Zb;
   
Xi1 = Xb'*s - 2*cd*Wy - c*Wx*Wz;
Xi2 = -Yb'*s - 2*cd*Wx + c*Wy*Wz;
Xi3 = yawddc*Xc'*Xb + 2*yawdc*Wz*Xc'*Yb - 2*yawdc*Wy*Xc'*Zb - Wx*Wy*Yc'*Yb - Wx*Wz*Yc'*Zb;

Wxd = B1*C3*Xi2/(A2*B1*C3);
Wyd = Xi1/B1;
Wzd = (B1*Xi3 - B3*Xi1)/(B1*C3);

Omega_d = [Wxd;Wyd;Wzd];

== matlab function suspend_kamotu_kato3/integrator1/MATLAB Function2 ==
  data: W input; Euler_angle_rate output; RPY input
function Euler_angle_rate = fcn(W, RPY)
roll = RPY(1);
pitch = RPY(2);
yaw = RPY(3);
rollS = sin(roll); rollC = cos(roll);           
pitchS = sin(pitch); pitchC = cos(pitch);       


Euler_angle_rate = pinv([1 0 -pitchS;
     0 rollC  pitchC * rollS;
     0 -rollS pitchC * rollC]) * W;

== matlab function suspend_kamotu_kato3/quadrotor position controller/MATLAB Function8 ==
  data: ex input; ev input; x_dd input; R input; F output; f output
function [F, f]= fcn(ex,ev,x_dd,R)
p = paramdef;
m = p.mQ;
e3 = [0;0;1];

ex_x = p.kp(1)*ex(1);
ex_y = p.kp(2)*ex(2);
ex_z = p.kp(3)*ex(3);
ex_d = [ex_x; ex_y; ex_z];

ev_x = p.kpd(1)*ev(1);
ev_y = p.kpd(2)*ev(2);
ev_z = p.kpd(3)*ev(3);
ev_d = [ev_x; ev_y; ev_z];
 
u = dot(ex_d + ev_d + m*x_dd, R*e3);
F = ex_d + ev_d + m*x_dd;

f = u;

== matlab function suspend_kamotu_kato3/Subsystem/Quadrotor Dynamics ==
  data: F input; M input; R input; wd input; Q_Pdd output; Omega_d output
function [Q_Pdd,Omega_d] = fcn(F, M, R, wd)
p = paramdef;
f = dot(F, R*p.e3);
Q_Pdd = (f*R*p.e3/p.mQ) - p.g*p.e3;
Omega_d = pinv(p.I)*(M - cross(wd, p.I*wd));

== matlab function suspend_kamotu_kato3/reference trajectory/Reference Trajectory ==
  data: ref_X output; ref_Vb output; ref_Accb output; ref_jarkb output; ref_snapb output; t input; T input; r input; ref_Yaw output; ref_Yawd output; ref_Yawdd output
function [ref_X, ref_Vb, ref_Accb, ref_jarkb, ref_snapb, ref_Yaw, ref_Yawd, ref_Yawdd] = fcn(t,T,r)
% 軌道生成
w = 2 * pi/T;          % 角周波数

% 中心　半径　　
c = [0;0;0];

ref_X = c + r*[sin(w*t); cos(w*t); 0];
ref_Vb = r*[w*cos(w*t); -w*sin(w*t); 0];
ref_Accb = [-r*w^2*sin(w*t); -r*w^2*cos(w*t); 9.8];
ref_jarkb = r*[-w^3*cos(w*t); w^3*sin(w*t); 0];
ref_snapb = r*[w^4*sin(w*t); w^4*cos(w*t); 0];

ref_X = c + r*[0; 0; 0];
ref_Vb = r*[0; 0; 100];
ref_Accb = [0; 0; 9.8];
ref_jarkb = r*[0;0; 0];
ref_snapb = r*[0;0; 0];

ref_X = c + r*[sin(w*t); 0; 0];
ref_Vb = r*[w*cos(w*t); 0; 0];
ref_Accb = [-r*w^2*sin(w*t); 0; 9.8];
ref_jarkb = r*[-w^3*cos(w*t); 0; 0];
ref_snapb = r*[w^4*sin(w*t); 0; 0];

ref_Yaw = 0;
ref_Yawd = 0;
ref_Yawdd = 0;

== matlab function suspend_kamotu_kato3/quadrotor attitude controller/calculate desired augular acceleration ==
  data: j input; s input; F input; Omega_d output; Rc input; Omega_c input; yawc input; yawdc input; yawddc input
function Omega_d = fcn(j, s, F,Rc, Omega_c, yawc, yawdc, yawddc)
p = paramdef;
m = p.mQ;
Xc = [cos(yawc); sin(yawc); 0];
Yc = [-sin(yawc); cos(yawc); 0];

Zw = [0;0;1];
Xb = Rc(:, 1);
Yb = Rc(:, 2);
Zb = Rc(:, 3);

Wx = Omega_c(3, 2);
Wy = Omega_c(1, 3);
Wz = Omega_c(2, 1);

c =  Zb'*F;
cd = (Rc*Omega_c*Zw)' * F + Zb'*j;

B1 = c;
C3 = norm(cross(Yc, Zb));
A2 = c;
B3 = -Yc'*Zb;
   
Xi1 = Xb'*s - 2*cd*Wy - c*Wx*Wz;
Xi2 = -Yb'*s - 2*cd*Wx + c*Wy*Wz;
Xi3 = yawddc*Xc'*Xb + 2*yawdc*Wz*Xc'*Yb - 2*yawdc*Wy*Xc'*Zb - Wx*Wy*Yc'*Yb - Wx*Wz*Yc'*Zb;

Wxd = B1*C3*Xi2/(A2*B1*C3);
Wyd = Xi1/B1;
Wzd = (B1*Xi3 - B3*Xi1)/(B1*C3);

Omega_d = [Wxd;Wyd;Wzd];

== matlab function suspend_kamotu_kato3/quadrotor attitude controller/calcurate desired attitude ==
  data: F input; Rc output; yawc input
function Rc = fcn(F, yawc)

b3c = F/norm(F);
c1c = [cos(yawc); sin(yawc); 0];
c2c = [-sin(yawc); cos(yawc); 0];

b1c = cross(cross(b3c, c1c)/norm(cross(b3c, c1c)), b3c);
b2c = cross(b3c, c1c)/norm(cross(b3c, c1c));
Rc = [b1c'; b2c'; b3c'];

== matlab function suspend_kamotu_kato3/quadrotor attitude controller/input Moment ==
  data: eR input; R input; Rc input; eOmega input; Omega input; Omega_c input; Omega_dc input; M output
function M = fcn(eR, R, Rc, eOmega, Omega, Omega_c, Omega_dc)

p = paramdef;
Omegavee = [0 -Omega(3) Omega(2); Omega(3) 0 -Omega(1); -Omega(2) Omega(1) 0];
% 角速度入力の時
% M = -p.kR*eR + Omega_c; %- p.I*(cross(Omegavee, R'*Rc*Omega_c) - R'*Rc*Omega_d);

% トルク入力の時
M = -p.kR*eR - p.kOmega*eOmega + cross(Omega, p.I*Omega) - p.I*(Omegavee*R'*Rc*Omega_c - R'*Rc*Omega_dc);
% M = -p.kR*eR - p.kOmega*eOmega + p.I*Omega_dc;

== matlab function suspend_kamotu_kato3/Subsystem1/cal PID payload Err/Payload Position1 ==
  data: drone_x input; xL output; cablevec input; cablevec_velocity input; velocity input; xL_d output
function [xL,xL_d] = fcn(drone_x,cablevec,cablevec_velocity,velocity)
p = paramdef;
xL = drone_x + p.L * cablevec;
xL_d = velocity + p.L * cablevec_velocity;

== matlab function suspend_kamotu_kato3/Subsystem2/Quadrotor Dynamics ==
  data: f input; M input; R input; wd input; Q_Pdd output; Omega_d output
function [Q_Pdd,Omega_d] = fcn(f, M, R, wd)
p = paramdef;
Q_Pdd = (f*R*p.e3/p.mQ) - p.g*p.e3;
Omega_d = pinv(p.I)*(M - cross(wd, p.I*wd));
% Omega_d = pinv(p.I)*(M);

== matlab function suspend_kamotu_kato3/integrator1/MATLAB Function ==
  data: R input; Rd output; Wb input
function Rd = fcn(R, Wb)
wx = Wb(1);
wy = Wb(2);
wz = Wb(3);
Wb = [ 0    -wz   wy;
       wz    0   -wx;
      -wy    wx   0];
Rd = R * Wb;

== matlab function suspend_kamotu_kato3/integrator1/acc 2 vec ==
  data: xL_dd input; P output
function P  = fcn(xL_dd)                 
g = 9.8;
P = -(xL_dd + g * [0;0;1])/norm(xL_dd + g * [0;0;1]);%ケーブルベクトル

== matlab function suspend_kamotu_kato3/Subsystem/Payload dynamics ==
  data: F input; R input; P input; xL_dd output; P_d input; Pdd output
function [xL_dd, Pdd]  = fcn(F,R,P,P_d)                 
g = 9.8;
e3 = [0;0;1];
p = paramdef;
f = dot(F, R*p.e3);
xL_dd = (P'*f*R*e3 -p.mQ*p.L*(dot(P_d,P_d))*P)/(p.mQ + p.mL) - g*e3;
Pdd = cross(P, cross(P, f*R*e3))/(p.mQ*p.L)-dot(P_d, P_d)*P;

== matlab function suspend_kamotu_kato3/quadrotor attitude controller1/Angular Velocity Error ==
  data: Rc input; Omega input; R input; Omega_c input; eOmega output
function eOmega = fcn(Rc, Omega,R, Omega_c)

eOmega = Omega - R'*Rc*Omega_c;
% eOmega = Omega - Omega_c;

== matlab function suspend_kamotu_kato3/quadrotor attitude controller1/Rotation Matrics Error ==
  data: Rc input; R input; eR output
function eR = fcn(Rc, R)

eR = (Rc'*R - R'*Rc)/2;

== matlab function suspend_kamotu_kato3/quadrotor attitude controller1/calculate desired angular veocity ==
  data: F input; Omega_c output; Rc input; yawc input; yawdc input; jarkc input
function Omega_c = fcn(F, Rc, yawc, yawdc, jarkc)

b1c = zeros(3, 1);b2c = zeros(3, 1);b3c = zeros(3, 1);

b1c = Rc(:, 1);
b2c = Rc(:, 2);

b3c = F/norm(F);
c1c = [cos(yawc); sin(yawc); 0];
c2c = [-sin(yawc) cos(yawc) 0]';

wy = dot(b1c, jarkc) / dot(b3c, F);
wx = - dot(b2c, jarkc) / dot(b3c, F);
wz = (yawdc * dot(c1c, b1c) + wy * dot(c2c, b3c))/norm(cross(c2c, b3c));

ref_W = [wx wy wz];
Omega_c = [0,-wz,wy; wz,0,-wx; -wy,wx,0];
